simulink subsystem "Linearized_discrete_drone_plant"  (R2020a)
settings: Solver=VariableStepAuto  StartTime=0.0  StopTime=10.0  RelTol=1e-3
undefined symbols (not defined in the file or in its folder): DiscIntNeverNeededParam
settings Model: Creator=augus  LastModifiedBy=augus

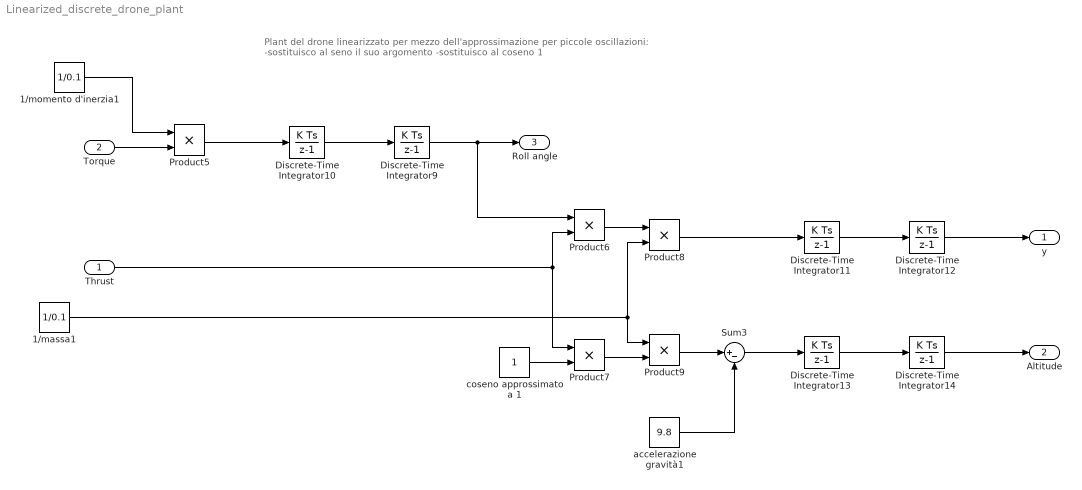
== system Linearized_discrete_drone_plant ==
  note: Plant del drone linearizzato per mezzo dell'approssimazione per piccole oscillazioni:
      | -sostituisco al seno il suo argomento
      | -sostituisco al coseno 1
  Thrust : Inport  Tag=tau
  Torque : Inport  Port=2
  1/massa1 : Constant  Value=1/0.1
  1/momento d'inerzia1 : Constant  Value=1/0.1
  Discrete-Time Integrator{9..14} (6 alike) : DiscreteIntegrator  SampleTime=-1  ICPrevOutput=DiscIntNeverNeededParam  ICPrevScaledInput=DiscIntNeverNeededParam
  Product{5..9} (5 alike) : Product
  Sum3 : Sum  Inputs=|+-
  accelerazione gravità1 : Constant  Value=9.8
  coseno approssimato a 1 : Constant
  y : Outport
  Altitude : Outport  Port=2
  Roll angle : Outport  Port=3
  wires:
  Product8/1 -> Discrete-Time Integrator11/1
  Product5/1 -> Discrete-Time Integrator10/1
  1/massa1/1 -> Product9/1, Product8/2
  1/momento d'inerzia1/1 -> Product5/1
  Discrete-Time Integrator11/1 -> Discrete-Time Integrator12/1
  accelerazione gravità1/1 -> Sum3/2
  Product7/1 -> Product9/2
  Product9/1 -> Sum3/1
  Discrete-Time Integrator10/1 -> Discrete-Time Integrator9/1
  Product6/1 -> Product8/1
  coseno approssimato a 1/1 -> Product7/2
  Discrete-Time Integrator13/1 -> Discrete-Time Integrator14/1
  Sum3/1 -> Discrete-Time Integrator13/1
  Thrust/1 -> Product7/1, Product6/2
  Discrete-Time Integrator9/1 -> Roll angle/1, Product6/1
  Discrete-Time Integrator14/1 -> Altitude/1
  Discrete-Time Integrator12/1 -> y/1
  Torque/1 -> Product5/2
